simulink model "Continuous_Dc_Motor_Model"  (R2024a)
settings: Solver=ode23s  StartTime=0.0  StopTime=10.0
model workspace (MAT data in the model file):
  J = 5e-05
  K = 0.2
  L = 0.01
  R = 4
  Ts = 0.01
  V = 7.4
  a1 = 0.5
  a2 = 2
  a3 = 2.5
  b = 5e-05
  ki = 7.33
  kp = 10
settings Model: Creator=BIDO  LastModifiedBy=BIDO

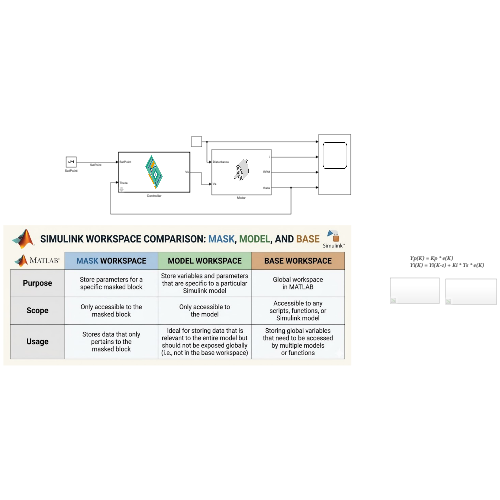
[thumbnail: Simulink's stored preview of the top-level diagram]
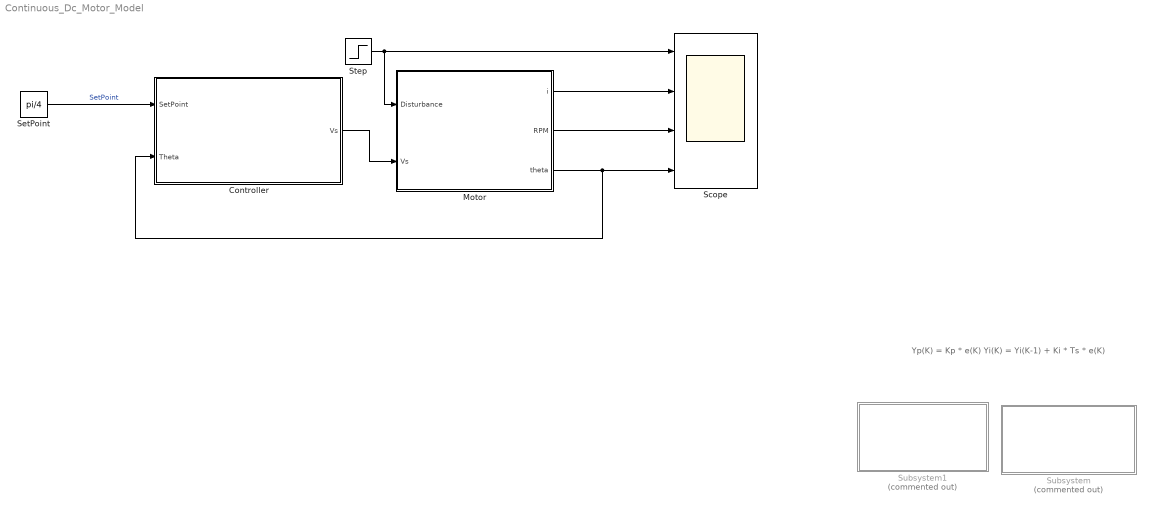
== system Continuous_Dc_Motor_Model ==
  note: Yp(K) = Kp * e(K)
      | Yi(K) = Yi(K-1) + Ki * Ts * e(K)
  Controller : Subsystem  TreatAsAtomicUnit=on  mask{kp=9.39, ki=7.33, Ts=0.01}
      mask prompts: kp "Propotional Gain"; ki "Integral Gain"; Ts "Sample time"
      mask Display: image('controller.PNG');
  Motor : Subsystem
      mask Display: image('DCmotor.PNG');
  Scope : Scope  NumInputPorts=4
  SetPoint : Constant  Value=pi/4
  Step : Step  After=0.1  SampleTime=0
  Subsystem : Subsystem  Commented=on
  Subsystem1 : Subsystem  Commented=on
  wires:
  Motor/3(theta) -> Scope/4, Controller/2(Theta)
  Motor/1(i) -> Scope/2
  Motor/2(RPM) -> Scope/3
  SetPoint/1 -> Controller/1(SetPoint)  "SetPoint"
  Controller/1(Vs) -> Motor/2(Vs)
  Step/1 -> Motor/1(Disturbance), Scope/1

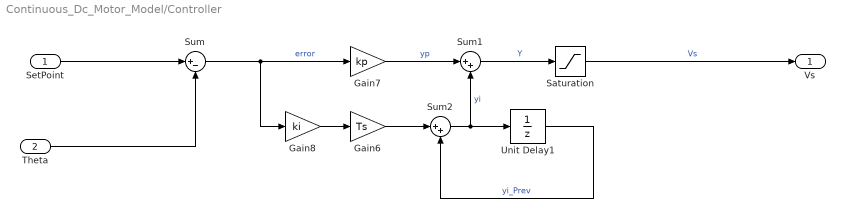
== system Continuous_Dc_Motor_Model/Controller ==
  SetPoint : Inport
  Theta : Inport  Port=2
  Gain6 : Gain  Gain=Ts
  Gain7 : Gain  Gain=kp
  Gain8 : Gain  Gain=ki
  Saturation : Saturate  UpperLimit=V  LowerLimit=-V
  Sum : Sum  Inputs=|+-
  Sum1 : Sum  Inputs=|++
  Sum2 : Sum  Inputs=|++
  Unit Delay1 : UnitDelay  SampleTime=Ts  HasFrameUpgradeWarning=on
  Vs : Outport
  wires:
  Sum1/1 -> Saturation/1  "Y"
  Gain7/1 -> Sum1/1  "yp"
  Unit Delay1/1 -> Sum2/2  "yi_Prev"
  Theta/1 -> Sum/2
  Sum2/1 -> Sum1/2, Unit Delay1/1  "yi"
  Gain8/1 -> Gain6/1
  Gain6/1 -> Sum2/1
  Sum/1 -> Gain8/1, Gain7/1  "error"
  SetPoint/1 -> Sum/1
  Saturation/1 -> Vs/1  "Vs"

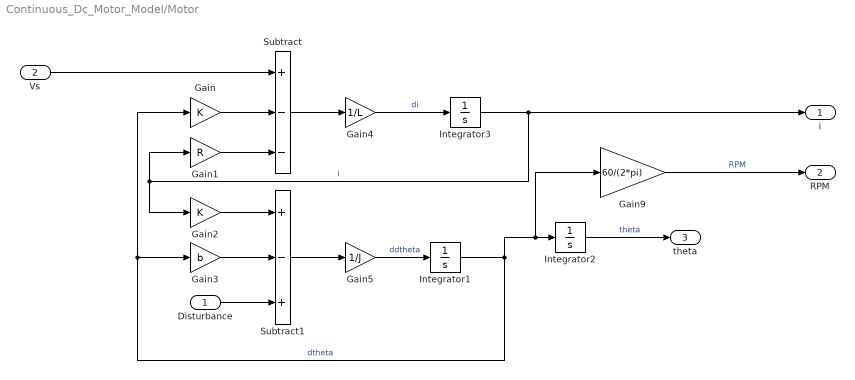
== system Continuous_Dc_Motor_Model/Motor ==
  Disturbance : Inport
  Vs : Inport  Port=2
  Gain : Gain  Gain=K
  Gain1 : Gain  Gain=R
  Gain2 : Gain  Gain=K
  Gain3 : Gain  Gain=b
  Gain4 : Gain  Gain=1/L
  Gain5 : Gain  Gain=1/J
  Gain9 : Gain  Gain=60/(2*pi)
  Integrator1 : Integrator  ContinuousStateAttributes='Velocity'
  Integrator2 : Integrator  ZeroCross=off  ContinuousStateAttributes='Angle'
  Integrator3 : Integrator
  Subtract : Sum  Inputs=+--
  Subtract1 : Sum  Inputs=+-+
  i : Outport
  RPM : Outport  Port=2
  theta : Outport  Port=3
  wires:
  Subtract/1 -> Gain4/1
  Integrator1/1 -> Gain9/1, Integrator2/1, Gain3/1, Gain/1  "dtheta"
  Gain3/1 -> Subtract1/2
  Gain/1 -> Subtract/2
  Integrator3/1 -> i/1, Gain1/1, Gain2/1  "i"
  Subtract1/1 -> Gain5/1
  Gain1/1 -> Subtract/3
  Gain4/1 -> Integrator3/1  "di"
  Gain2/1 -> Subtract1/1
  Gain5/1 -> Integrator1/1  "ddtheta"
  Vs/1 -> Subtract/1
  Gain9/1 -> RPM/1  "RPM"
  Integrator2/1 -> theta/1  "theta"
  Disturbance/1 -> Subtract1/3

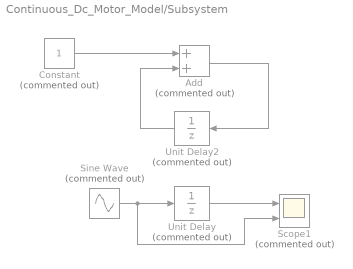
== system Continuous_Dc_Motor_Model/Subsystem ==
  Add : Sum  Commented=on
  Constant : Constant  Commented=on
  Scope1 : Scope  Commented=on  NumInputPorts=2
  Sine Wave : Sin  Commented=on  Phase=pi/2  SampleTime=0.4
  Unit Delay : UnitDelay  Commented=on  SampleTime=0.8  HasFrameUpgradeWarning=on
  Unit Delay2 : UnitDelay  Commented=on  HasFrameUpgradeWarning=on
  wires:
  Unit Delay/1 -> Scope1/1
  Unit Delay2/1 -> Add/2
  Sine Wave/1 -> Unit Delay/1, Scope1/2
  Add/1 -> Unit Delay2/1
  Constant/1 -> Add/1

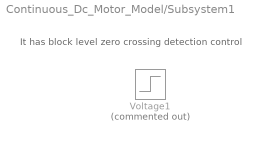
== system Continuous_Dc_Motor_Model/Subsystem1 ==
  note: It has block level zero crossing detection control
  Voltage1 : Step  Commented=on  After=V  SampleTime=0
